simulink model "rThrottle"  (R2024b)
settings: configuration reference "STM32H7_Config" (kept outside this file)
undefined symbols (not defined in the file): rThrottleCalHigh, rThrottleCalLow, VThrottle1HighSample, VThrottle1LowSample, VThrottle2HighSample, VThrottle2LowSample
settings Model: DataDictionary=Master_Dictionary.sldd  EnableAccessToBaseWorkspace=off  Creator=torni  LastModifiedBy=William
settings ConfigSetRef: SourceName=STM32H7_Config

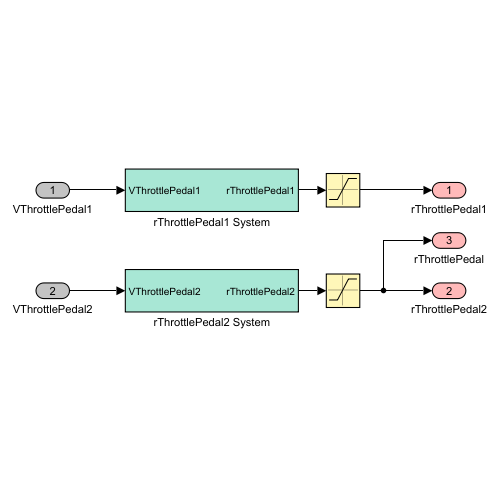
[thumbnail: Simulink's stored preview of the top-level diagram]
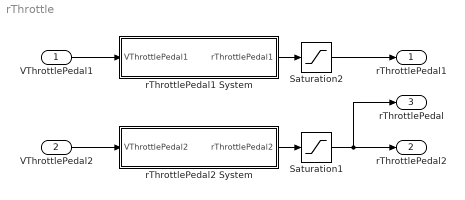
== system rThrottle ==
  VThrottlePedal1 : Inport  OutDataTypeStr=double
  VThrottlePedal2 : Inport  Port=2  OutDataTypeStr=double
  Saturation1 : Saturate  UpperLimit=100  LowerLimit=0
  Saturation2 : Saturate  UpperLimit=100  LowerLimit=0
  rThrottlePedal1 System : Subsystem
  rThrottlePedal2 System : Subsystem
  rThrottlePedal1 : Outport  OutDataTypeStr=double  VectorParamsAs1DForOutWhenUnconnected=off
  rThrottlePedal2 : Outport  Port=2  OutDataTypeStr=double  VectorParamsAs1DForOutWhenUnconnected=off
  rThrottlePedal : Outport  Port=3  OutDataTypeStr=double  VectorParamsAs1DForOutWhenUnconnected=off
  wires:
  rThrottlePedal1 System/1(rThrottlePedal1) -> Saturation2/1
  VThrottlePedal1/1 -> rThrottlePedal1 System/1(VThrottlePedal1)
  VThrottlePedal2/1 -> rThrottlePedal2 System/1(VThrottlePedal2)
  rThrottlePedal2 System/1(rThrottlePedal2) -> Saturation1/1
  Saturation2/1 -> rThrottlePedal1/1
  Saturation1/1 -> rThrottlePedal2/1, rThrottlePedal/1

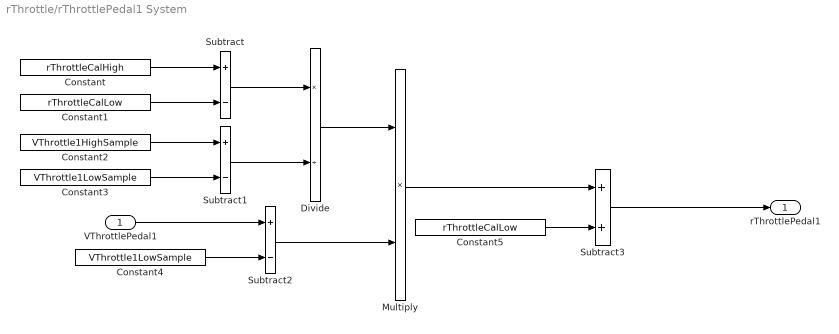
== system rThrottle/rThrottlePedal1 System ==
  VThrottlePedal1 : Inport  OutDataTypeStr=double
  Constant : Constant  Value=rThrottleCalHigh
  Constant1 : Constant  Value=rThrottleCalLow
  Constant2 : Constant  Value=VThrottle1HighSample
  Constant3 : Constant  Value=VThrottle1LowSample
  Constant4 : Constant  Value=VThrottle1LowSample
  Constant5 : Constant  Value=rThrottleCalLow
  Divide : Product  Inputs=*/
  Multiply : Product
  Subtract : Sum  Inputs=+-
  Subtract1 : Sum  Inputs=+-
  Subtract2 : Sum  Inputs=+-
  Subtract3 : Sum
  rThrottlePedal1 : Outport  OutDataTypeStr=double  VectorParamsAs1DForOutWhenUnconnected=off
  wires:
  VThrottlePedal1/1 -> Subtract2/1
  Subtract1/1 -> Divide/2
  Constant4/1 -> Subtract2/2
  Constant5/1 -> Subtract3/2
  Divide/1 -> Multiply/1
  Subtract3/1 -> rThrottlePedal1/1
  Constant3/1 -> Subtract1/2
  Multiply/1 -> Subtract3/1
  Constant/1 -> Subtract/1
  Constant2/1 -> Subtract1/1
  Subtract2/1 -> Multiply/2
  Subtract/1 -> Divide/1
  Constant1/1 -> Subtract/2

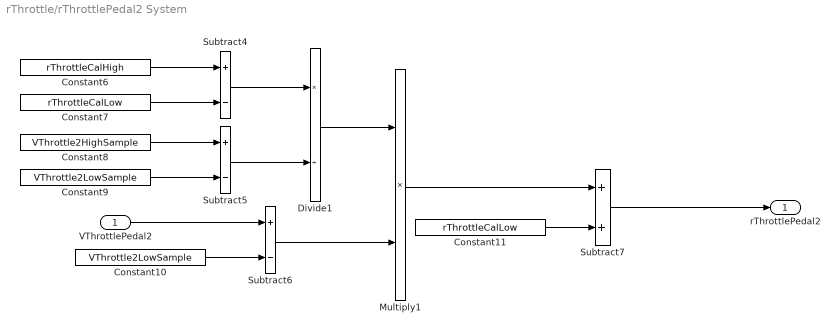
== system rThrottle/rThrottlePedal2 System ==
  VThrottlePedal2 : Inport  OutDataTypeStr=double
  Constant10 : Constant  Value=VThrottle2LowSample
  Constant11 : Constant  Value=rThrottleCalLow
  Constant6 : Constant  Value=rThrottleCalHigh
  Constant7 : Constant  Value=rThrottleCalLow
  Constant8 : Constant  Value=VThrottle2HighSample
  Constant9 : Constant  Value=VThrottle2LowSample
  Divide1 : Product  Inputs=*/
  Multiply1 : Product
  Subtract4 : Sum  Inputs=+-
  Subtract5 : Sum  Inputs=+-
  Subtract6 : Sum  Inputs=+-
  Subtract7 : Sum
  rThrottlePedal2 : Outport  OutDataTypeStr=double  VectorParamsAs1DForOutWhenUnconnected=off
  wires:
  Subtract6/1 -> Multiply1/2
  Constant9/1 -> Subtract5/2
  Constant8/1 -> Subtract5/1
  Constant10/1 -> Subtract6/2
  Divide1/1 -> Multiply1/1
  Constant6/1 -> Subtract4/1
  Subtract5/1 -> Divide1/2
  Constant11/1 -> Subtract7/2
  Subtract4/1 -> Divide1/1
  Constant7/1 -> Subtract4/2
  Subtract7/1 -> rThrottlePedal2/1
  VThrottlePedal2/1 -> Subtract6/1
  Multiply1/1 -> Subtract7/1
